simulink model "closed_loop_example"  (R2020b)
settings: Solver=VariableStepDiscrete  StartTime=0.0  StopTime=1000  FixedStep=.01  MaxStep=0.2  MinStep=0.01  RelTol=1e-3
settings Model: EnablePacing=on  Creator=celit  LastModifiedBy=celit
settings SolverCC: ZeroCrossAlgorithm=Adaptive
settings SFSimCC: SimCustomHeaderCode="#include \"mono_src/my_func1.h\""  SimUserSources=mono_src/my_func1.cpp  SimUserIncludeDirs=mono_src  SimParseCustomCode=off  CustomCodeUndefinedFunction=UseInterfaceOnly

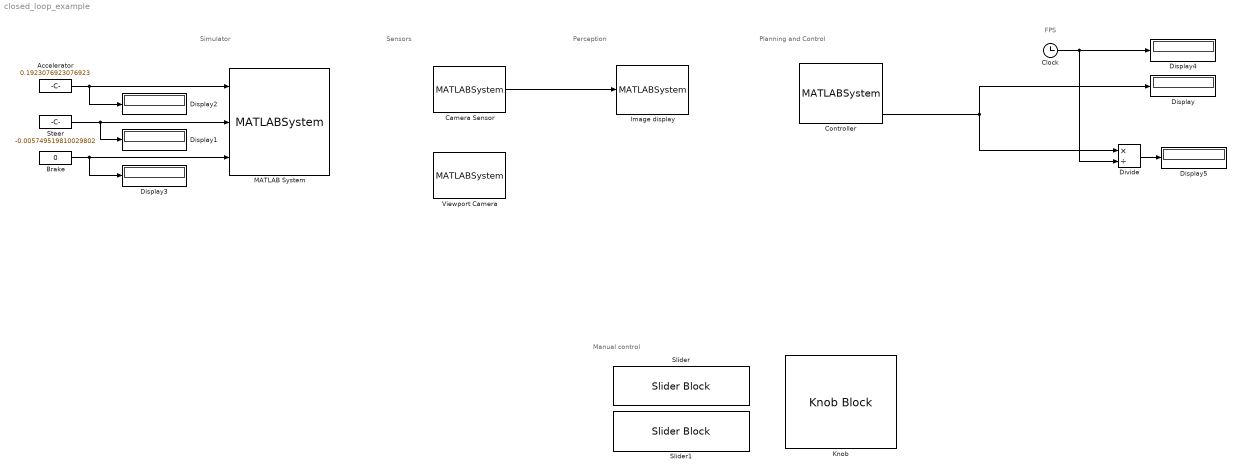
== system closed_loop_example ==
  note: Sensors
  note: Simulator
  note: FPS
  note: Perception
  note: Planning and Control
  note: Manual control
  Accelerator : Constant  Value=0.1923076923076923  OutDataTypeStr=double  SampleTime=-1
  Brake : Constant  Value=0  OutDataTypeStr=double  SampleTime=-1
  Camera Sensor : MATLABSystem  Priority=1  System=Camera  config_path=configurations/camera.json  SimulateUsing=Interpreted execution
      mask Type: Camera
      mask Display:
      | disp('Camera');
      | port_label('output',1,'y');
  Clock : Clock
  Controller : MATLABSystem  Priority=3  System=VehicleController  Kp=1.0  Ki=0.0  Kd=0.0  SimulateUsing=Interpreted execution
      mask Type: VehicleController
      mask Display:
      | disp('VehicleController');
      | port_label('input',1,'x');
      | port_label('output',1,'forward');
      | port_label('output',2,'right');
      | port_label('output',3,'brake');
      | port_label('output',4,'count');
  Display{,1..5} (6 alike) : Display
  Divide : Product  Inputs=*/
  Image display : MATLABSystem  Priority=2  System=Perception  draw_annotations=false  SimulateUsing=Interpreted execution
      mask Type: Perception
      mask Display:
      | disp('Perception');
      | port_label('input',1,'image');
  Knob : KnobBlock  LabelPosition=Bottom  ScaleMin=-1  ScaleMax=1  TickInterval=.25
  MATLAB System : MATLABSystem  Priority=0  System=Simulator  sim_config_path=configurations/simulator.json  scenario_config_path=configurations/trajectories/scenario_config_single_vehicle.json  weather_config_path=configurations/weather.json  server_ip=127.0.0.1  server_port=8999  SampleTime=0.333  OffsetTime=0.0  TickTime=0.1  SimulateUsing=Interpreted execution
      mask Type: Simulator
      mask Display:
      | disp('Simulator');
      | port_label('input',1,'forward');
      | port_label('input',2,'right');
      | port_label('input',3,'brake');
  Slider : SliderBlock  LabelPosition=Bottom  ScaleMax=1  TickInterval=.2
  Slider1 : SliderBlock  LabelPosition=Bottom  ScaleMax=1  TickInterval=.2
  Steer : Constant  Value=-0.005749519810029802  SampleTime=-1
  Viewport Camera : MATLABSystem  Priority=1  System=ViewportCamera  config_path=configurations/viewport_camera.json  SimulateUsing=Interpreted execution
      mask Type: ViewportCamera
      mask Display:
      | disp('ViewportCamera');
      | port_label('output',1,'y');
  wires:
  Accelerator/1 -> Display2/1, MATLAB System/1
  Brake/1 -> Display3/1, MATLAB System/3
  Steer/1 -> Display1/1, MATLAB System/2
  Clock/1 -> Divide/2, Display4/1
  Divide/1 -> Display5/1
  Controller/4 -> Divide/1, Display/1
  Camera Sensor/1 -> Image display/1
